simulink model "DEF_IEEE14"  (R2022b)
settings: Solver=FixedStepAuto  StartTime=0  StopTime=15  FixedStep=Ts  RelTol=1e-3
undefined symbols (not defined in the file or in its folder): ApparatusDiscreDamping, ApparatusPara, ApparatusPowerFlow, ApparatusType, Fbase, OtherInputs, Sbase, Ts, Vbase, Wbase, x_e, Ybase, Zbase
libraries: spsGroundLib x22, SimplusGT x22, spsThreePhaseSeriesRLCBranchLib x20, spsThreePhaseParallelRLCBranchLib x14, spsabctoAlphaBetaZeroLib x4, spsThreePhaseTransformerTwoWindingsLib x3, spspowerguiLib x1
settings Model: Creator=y_zhu  LastModifiedBy=yz34218

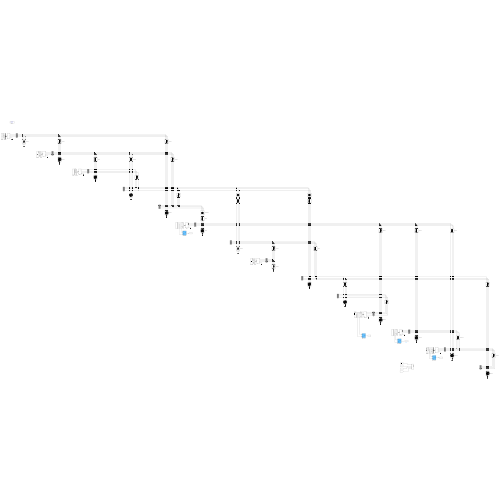
[thumbnail: Simulink's stored preview of the top-level diagram]
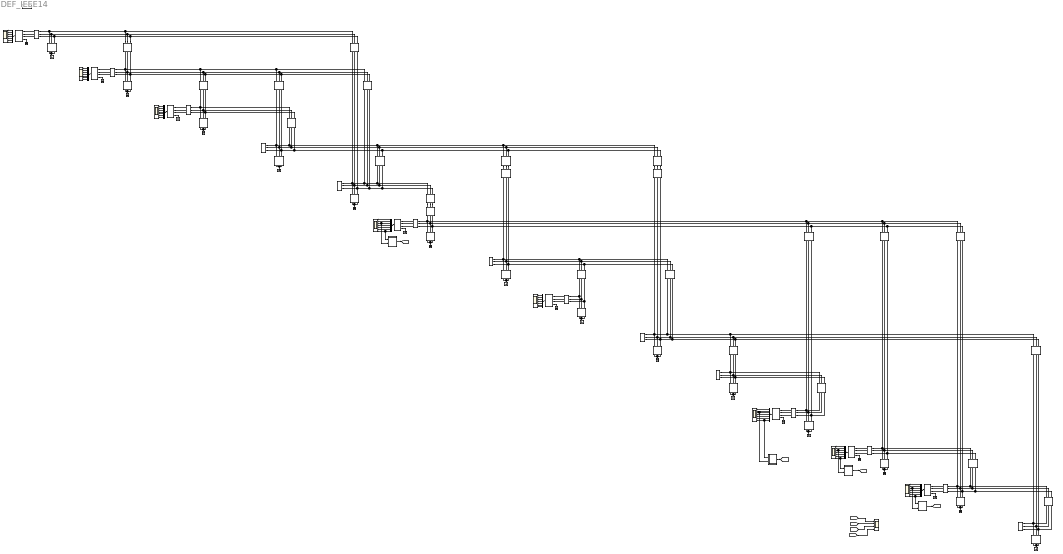
== system DEF_IEEE14 ==
  B-GND{1,4,8,10,14,16,20,23..24,27,29..30,32,34} (14 alike) : spsGroundLib/Ground  LConnTagsString=a
  Branch1-1 : spsThreePhaseParallelRLCBranchLib/Three-Phase Parallel RLC Branch  LConnTagsString=A|B|C  RConnTagsString=A|B|C  BranchType=C  Resistance=(Inf)*Zbase  Inductance=(Inf)*Zbase/Wbase  Capacitance=(0.051)*Ybase/Wbase  Measurements=None
  Branch1-2 : spsThreePhaseSeriesRLCBranchLib/Three-Phase Series RLC Branch  LConnTagsString=A|B|C  RConnTagsString=A|B|C  BranchType=RL  Resistance=(0.01938)*Zbase  Inductance=(0.05917)*Zbase/Wbase  Capacitance=1e-6  Measurements=None
  Branch1-5 : spsThreePhaseSeriesRLCBranchLib/Three-Phase Series RLC Branch  LConnTagsString=A|B|C  RConnTagsString=A|B|C  BranchType=RL  Resistance=(0.05403)*Zbase  Inductance=(0.22304)*Zbase/Wbase  Capacitance=1e-6  Measurements=None
  Branch10-10 : spsThreePhaseParallelRLCBranchLib/Three-Phase Parallel RLC Branch  LConnTagsString=A|B|C  RConnTagsString=A|B|C  BranchType=RLC  Resistance=(12.2907)*Zbase  Inductance=(19.0718)*Zbase/Wbase  Capacitance=(1e-07)*Ybase/Wbase  Measurements=None
  Branch10-11 : spsThreePhaseSeriesRLCBranchLib/Three-Phase Series RLC Branch  LConnTagsString=A|B|C  RConnTagsString=A|B|C  BranchType=RL  Resistance=(0.08205)*Zbase  Inductance=(0.19207)*Zbase/Wbase  Capacitance=1e-6  Measurements=None
  Branch11-11 : spsThreePhaseParallelRLCBranchLib/Three-Phase Parallel RLC Branch  LConnTagsString=A|B|C  RConnTagsString=A|B|C  BranchType=RLC  Resistance=(10.675)*Zbase  Inductance=(62.2711)*Zbase/Wbase  Capacitance=(1e-07)*Ybase/Wbase  Measurements=None
  Branch12-12 : spsThreePhaseParallelRLCBranchLib/Three-Phase Parallel RLC Branch  LConnTagsString=A|B|C  RConnTagsString=A|B|C  BranchType=RLC  Resistance=(6.03)*Zbase  Inductance=(68.9685)*Zbase/Wbase  Capacitance=(1e-07)*Ybase/Wbase  Measurements=None
  Branch12-13 : spsThreePhaseSeriesRLCBranchLib/Three-Phase Series RLC Branch  LConnTagsString=A|B|C  RConnTagsString=A|B|C  BranchType=RL  Resistance=(0.22092)*Zbase  Inductance=(0.19988)*Zbase/Wbase  Capacitance=1e-6  Measurements=None
  Branch13-13 : spsThreePhaseParallelRLCBranchLib/Three-Phase Parallel RLC Branch  LConnTagsString=A|B|C  RConnTagsString=A|B|C  BranchType=RLC  Resistance=(2.6813)*Zbase  Inductance=(18.7232)*Zbase/Wbase  Capacitance=(1.5e-07)*Ybase/Wbase  Measurements=None
  Branch13-14 : spsThreePhaseSeriesRLCBranchLib/Three-Phase Series RLC Branch  LConnTagsString=A|B|C  RConnTagsString=A|B|C  BranchType=RL  Resistance=(0.17093)*Zbase  Inductance=(0.34802)*Zbase/Wbase  Capacitance=1e-6  Measurements=None
  Branch14-14 : spsThreePhaseParallelRLCBranchLib/Three-Phase Parallel RLC Branch  LConnTagsString=A|B|C  RConnTagsString=A|B|C  BranchType=RLC  Resistance=(7.1477)*Zbase  Inductance=(21.3001)*Zbase/Wbase  Capacitance=(1e-07)*Ybase/Wbase  Measurements=None
  Branch2-2 : spsThreePhaseParallelRLCBranchLib/Three-Phase Parallel RLC Branch  LConnTagsString=A|B|C  RConnTagsString=A|B|C  BranchType=RLC  Resistance=(5.0324)*Zbase  Inductance=(8.5986)*Zbase/Wbase  Capacitance=(0.0826)*Ybase/Wbase  Measurements=None
  Branch2-3 : spsThreePhaseSeriesRLCBranchLib/Three-Phase Series RLC Branch  LConnTagsString=A|B|C  RConnTagsString=A|B|C  BranchType=RL  Resistance=(0.04699)*Zbase  Inductance=(0.19797)*Zbase/Wbase  Capacitance=1e-6  Measurements=None
  Branch2-4 : spsThreePhaseSeriesRLCBranchLib/Three-Phase Series RLC Branch  LConnTagsString=A|B|C  RConnTagsString=A|B|C  BranchType=RL  Resistance=(0.05811)*Zbase  Inductance=(0.17632)*Zbase/Wbase  Capacitance=1e-6  Measurements=None
  Branch2-5 : spsThreePhaseSeriesRLCBranchLib/Three-Phase Series RLC Branch  LConnTagsString=A|B|C  RConnTagsString=A|B|C  BranchType=RL  Resistance=(0.05695)*Zbase  Inductance=(0.17388)*Zbase/Wbase  Capacitance=1e-6  Measurements=None
  Branch3-3 : spsThreePhaseParallelRLCBranchLib/Three-Phase Parallel RLC Branch  LConnTagsString=A|B|C  RConnTagsString=A|B|C  BranchType=RLC  Resistance=(1.0829)*Zbase  Inductance=(5.3689)*Zbase/Wbase  Capacitance=(0.0283)*Ybase/Wbase  Measurements=None
  Branch3-4 : spsThreePhaseSeriesRLCBranchLib/Three-Phase Series RLC Branch  LConnTagsString=A|B|C  RConnTagsString=A|B|C  BranchType=RL  Resistance=(0.06701)*Zbase  Inductance=(0.17103)*Zbase/Wbase  Capacitance=1e-6  Measurements=None
  Branch4-4 : spsThreePhaseParallelRLCBranchLib/Three-Phase Parallel RLC Branch  LConnTagsString=A|B|C  RConnTagsString=A|B|C  BranchType=RC  Resistance=(2.1566)*Zbase  Inductance=(Inf)*Zbase/Wbase  Capacitance=(0.061233)*Ybase/Wbase  Measurements=None
  Branch4-5 : spsThreePhaseSeriesRLCBranchLib/Three-Phase Series RLC Branch  LConnTagsString=A|B|C  RConnTagsString=A|B|C  BranchType=RL  Resistance=(0.01335)*Zbase  Inductance=(0.04211)*Zbase/Wbase  Capacitance=1e-6  Measurements=None
  Branch4-7 : spsThreePhaseSeriesRLCBranchLib/Three-Phase Series RLC Branch  LConnTagsString=A|B|C  RConnTagsString=A|B|C  BranchType=RL  Resistance=(1e-07)*Zbase  Inductance=(0.20912)*Zbase/Wbase  Capacitance=1e-6  Measurements=None
  Branch4-9 : spsThreePhaseSeriesRLCBranchLib/Three-Phase Series RLC Branch  LConnTagsString=A|B|C  RConnTagsString=A|B|C  BranchType=RL  Resistance=(1e-07)*Zbase  Inductance=(0.55618)*Zbase/Wbase  Capacitance=1e-6  Measurements=None
  Branch5-5 : spsThreePhaseParallelRLCBranchLib/Three-Phase Parallel RLC Branch  LConnTagsString=A|B|C  RConnTagsString=A|B|C  BranchType=RLC  Resistance=(13.5986)*Zbase  Inductance=(64.5935)*Zbase/Wbase  Capacitance=(0.0419)*Ybase/Wbase  Measurements=None
  Branch5-6 : spsThreePhaseSeriesRLCBranchLib/Three-Phase Series RLC Branch  LConnTagsString=A|B|C  RConnTagsString=A|B|C  BranchType=RL  Resistance=(1e-07)*Zbase  Inductance=(0.25202)*Zbase/Wbase  Capacitance=1e-6  Measurements=None
  Branch6-11 : spsThreePhaseSeriesRLCBranchLib/Three-Phase Series RLC Branch  LConnTagsString=A|B|C  RConnTagsString=A|B|C  BranchType=RL  Resistance=(0.09498)*Zbase  Inductance=(0.1989)*Zbase/Wbase  Capacitance=1e-6  Measurements=None
  Branch6-12 : spsThreePhaseSeriesRLCBranchLib/Three-Phase Series RLC Branch  LConnTagsString=A|B|C  RConnTagsString=A|B|C  BranchType=RL  Resistance=(0.12291)*Zbase  Inductance=(0.25581)*Zbase/Wbase  Capacitance=1e-6  Measurements=None
  Branch6-13 : spsThreePhaseSeriesRLCBranchLib/Three-Phase Series RLC Branch  LConnTagsString=A|B|C  RConnTagsString=A|B|C  BranchType=RL  Resistance=(0.06615)*Zbase  Inductance=(0.13027)*Zbase/Wbase  Capacitance=1e-6  Measurements=None
  Branch6-6 : spsThreePhaseParallelRLCBranchLib/Three-Phase Parallel RLC Branch  LConnTagsString=A|B|C  RConnTagsString=A|B|C  BranchType=RLC  Resistance=(10.2223)*Zbase  Inductance=(15.2653)*Zbase/Wbase  Capacitance=(2e-07)*Ybase/Wbase  Measurements=None
  Branch7-7 : spsThreePhaseParallelRLCBranchLib/Three-Phase Parallel RLC Branch  LConnTagsString=A|B|C  RConnTagsString=A|B|C  BranchType=C  Resistance=(Inf)*Zbase  Inductance=(Inf)*Zbase/Wbase  Capacitance=(1.5e-07)*Ybase/Wbase  Measurements=None
  Branch7-8 : spsThreePhaseSeriesRLCBranchLib/Three-Phase Series RLC Branch  LConnTagsString=A|B|C  RConnTagsString=A|B|C  BranchType=RL  Resistance=(1e-07)*Zbase  Inductance=(0.17615)*Zbase/Wbase  Capacitance=1e-6  Measurements=None
  Branch7-9 : spsThreePhaseSeriesRLCBranchLib/Three-Phase Series RLC Branch  LConnTagsString=A|B|C  RConnTagsString=A|B|C  BranchType=RL  Resistance=(1e-07)*Zbase  Inductance=(0.11001)*Zbase/Wbase  Capacitance=1e-6  Measurements=None
  Branch8-8 : spsThreePhaseParallelRLCBranchLib/Three-Phase Parallel RLC Branch  LConnTagsString=A|B|C  RConnTagsString=A|B|C  BranchType=C  Resistance=(Inf)*Zbase  Inductance=(Inf)*Zbase/Wbase  Capacitance=(5e-08)*Ybase/Wbase  Measurements=None
  Branch9-10 : spsThreePhaseSeriesRLCBranchLib/Three-Phase Series RLC Branch  LConnTagsString=A|B|C  RConnTagsString=A|B|C  BranchType=RL  Resistance=(0.03181)*Zbase  Inductance=(0.0845)*Zbase/Wbase  Capacitance=1e-6  Measurements=None
  Branch9-14 : spsThreePhaseSeriesRLCBranchLib/Three-Phase Series RLC Branch  LConnTagsString=A|B|C  RConnTagsString=A|B|C  BranchType=RL  Resistance=(0.12711)*Zbase  Inductance=(0.27038)*Zbase/Wbase  Capacitance=1e-6  Measurements=None
  Branch9-9 : spsThreePhaseParallelRLCBranchLib/Three-Phase Parallel RLC Branch  LConnTagsString=A|B|C  RConnTagsString=A|B|C  BranchType=RLC  Resistance=(3.7813)*Zbase  Inductance=(6.7198)*Zbase/Wbase  Capacitance=(0.19)*Ybase/Wbase  Measurements=None
  Bus{1..14} (14 alike) : SimplusGT/Three-Phase Bus  Vbase=1  Sbase=1
  D-GND{1..3,6,8,11..13} (8 alike) : spsGroundLib/Ground  LConnTagsString=a
  D-Scope{1..3,6,8,11..13} (8 alike) : Scope  NumInputPorts=7
  DEF_Friction : Subsystem  mask{PowerFlow_App=ApparatusPowerFlow{11}}
      mask prompts: PowerFlow_App "Power Flow"
  DEF_Friction1 : Subsystem  mask{PowerFlow_App=ApparatusPowerFlow{12}}
      mask prompts: PowerFlow_App "Power Flow"
  DEF_Friction2 : Subsystem  mask{PowerFlow_App=ApparatusPowerFlow{13}}
      mask prompts: PowerFlow_App "Power Flow"
  DEF_Friction3 : Subsystem  mask{PowerFlow_App=ApparatusPowerFlow{6}}
      mask prompts: PowerFlow_App "Power Flow"
  DS-Bus{1..3,6,8,11..13} (8 alike) : BusSelector  OutputSignals=v_dq,i_dq,v_abc,i_abc,w,theta,pq
  SM1 : SimplusGT/SynchronousMachineFull_Cyp_SMAVRPSSGOV (dq-Frame System Object)  Ts=Ts  Sbase=Sbase  Vbase=Vbase  Wbase=Wbase  ApparatusType=ApparatusType{1}  ApparatusPara=ApparatusPara{1}  PowerFlow=ApparatusPowerFlow{1}  x0=x_e{1}  OtherInputs=OtherInputs{1}  DiscreMethod=Hybrid Trapezoidal  EnableInsideModification=off  DiscreDampingFlag=on  DiscreDampingValue=ApparatusDiscreDamping{1}  LinearizationTimes=1  DirectFeedthrough=off
  SM2 : SimplusGT/SynchronousMachineFull_Cyp_SMAVRPSSGOV (dq-Frame System Object)  Ts=Ts  Sbase=Sbase  Vbase=Vbase  Wbase=Wbase  ApparatusType=ApparatusType{2}  ApparatusPara=ApparatusPara{2}  PowerFlow=ApparatusPowerFlow{2}  x0=x_e{2}  OtherInputs=OtherInputs{2}  DiscreMethod=Hybrid Trapezoidal  EnableInsideModification=off  DiscreDampingFlag=on  DiscreDampingValue=ApparatusDiscreDamping{2}  LinearizationTimes=1  DirectFeedthrough=off
  SM3 : SimplusGT/SynchronousMachineFull_Cyp_SMAVR (dq-Frame System Object)  Ts=Ts  Sbase=Sbase  Vbase=Vbase  Wbase=Wbase  ApparatusType=ApparatusType{3}  ApparatusPara=ApparatusPara{3}  PowerFlow=ApparatusPowerFlow{3}  x0=x_e{3}  OtherInputs=OtherInputs{3}  DiscreMethod=Hybrid Trapezoidal  EnableInsideModification=off  DiscreDampingFlag=on  DiscreDampingValue=ApparatusDiscreDamping{3}  LinearizationTimes=1  DirectFeedthrough=off
  SM6 : SimplusGT/SynchronousMachineFull_Cyp_SMAVR (dq-Frame System Object)  Ts=Ts  Sbase=Sbase  Vbase=Vbase  Wbase=Wbase  ApparatusType=ApparatusType{6}  ApparatusPara=ApparatusPara{6}  PowerFlow=ApparatusPowerFlow{6}  x0=x_e{6}  OtherInputs=OtherInputs{6}  DiscreMethod=Hybrid Trapezoidal  EnableInsideModification=off  DiscreDampingFlag=on  DiscreDampingValue=ApparatusDiscreDamping{6}  LinearizationTimes=1  DirectFeedthrough=off
  SM8 : SimplusGT/SynchronousMachineFull_Cyp_SMAVR (dq-Frame System Object)  Ts=Ts  Sbase=Sbase  Vbase=Vbase  Wbase=Wbase  ApparatusType=ApparatusType{8}  ApparatusPara=ApparatusPara{8}  PowerFlow=ApparatusPowerFlow{8}  x0=x_e{8}  OtherInputs=OtherInputs{8}  DiscreMethod=Hybrid Trapezoidal  EnableInsideModification=off  DiscreDampingFlag=on  DiscreDampingValue=ApparatusDiscreDamping{8}  LinearizationTimes=1  DirectFeedthrough=off
  Scope : Scope  NumInputPorts=4
  Transformer4-7 : spsThreePhaseTransformerTwoWindingsLib/Three-Phase Transformer (Two Windings)  Winding1Connection=Yg  Winding2Connection=Yg  CoreType=Three single-phase transformers  SetSaturation=off  Hysteresis=off  DataFile='hysteresis'  SetInitialFlux=off  Measurements=None  UNITS=pu  NominalPower=[Sbase, Fbase]  Winding1=[0.978*Vbase, 0, 0]  Winding2=[Vbase, 0, 0]  Rm=1e4  Lm=1e4  L0=0.5  Saturation=[ 0,0 ; 0.0024,1.2 ; 1.0,1.52 ]  InitialFluxes=[ 0.8 , -0.8 , 0.7 ]  BreakLoop=off  DiscreteSolver=Trapezoidal iterative  DataType=off  TransfoNumber=1
  Transformer4-9 : spsThreePhaseTransformerTwoWindingsLib/Three-Phase Transformer (Two Windings)  Winding1Connection=Yg  Winding2Connection=Yg  CoreType=Three single-phase transformers  SetSaturation=off  Hysteresis=off  DataFile='hysteresis'  SetInitialFlux=off  Measurements=None  UNITS=pu  NominalPower=[Sbase, Fbase]  Winding1=[0.969*Vbase, 0, 0]  Winding2=[Vbase, 0, 0]  Rm=1e4  Lm=1e4  L0=0.5  Saturation=[ 0,0 ; 0.0024,1.2 ; 1.0,1.52 ]  InitialFluxes=[ 0.8 , -0.8 , 0.7 ]  BreakLoop=off  DiscreteSolver=Trapezoidal iterative  DataType=off  TransfoNumber=1
  Transformer5-6 : spsThreePhaseTransformerTwoWindingsLib/Three-Phase Transformer (Two Windings)  Winding1Connection=Yg  Winding2Connection=Yg  CoreType=Three single-phase transformers  SetSaturation=off  Hysteresis=off  DataFile='hysteresis'  SetInitialFlux=off  Measurements=None  UNITS=pu  NominalPower=[Sbase, Fbase]  Winding1=[0.932*Vbase, 0, 0]  Winding2=[Vbase, 0, 0]  Rm=1e4  Lm=1e4  L0=0.5  Saturation=[ 0,0 ; 0.0024,1.2 ; 1.0,1.52 ]  InitialFluxes=[ 0.8 , -0.8 , 0.7 ]  BreakLoop=off  DiscreteSolver=Trapezoidal iterative  DataType=off  TransfoNumber=1
  VSI-PLL11 : SimplusGT/Grid-Following Voltage-Source Inverter (dq-Frame System Object)  Ts=Ts  Sbase=Sbase  Vbase=Vbase  Wbase=Wbase  ApparatusType=ApparatusType{11}  ApparatusPara=ApparatusPara{11}  PowerFlow=ApparatusPowerFlow{11}  x0=x_e{11}  OtherInputs=OtherInputs{11}  DiscreMethod=Hybrid Trapezoidal  EnableInsideModification=off  DiscreDampingFlag=on  DiscreDampingValue=ApparatusDiscreDamping{11}  LinearizationTimes=1  DirectFeedthrough=off
  VSI-PLL12 : SimplusGT/Grid-Following Voltage-Source Inverter (dq-Frame System Object)  Ts=Ts  Sbase=Sbase  Vbase=Vbase  Wbase=Wbase  ApparatusType=ApparatusType{12}  ApparatusPara=ApparatusPara{12}  PowerFlow=ApparatusPowerFlow{12}  x0=x_e{12}  OtherInputs=OtherInputs{12}  DiscreMethod=Hybrid Trapezoidal  EnableInsideModification=off  DiscreDampingFlag=on  DiscreDampingValue=ApparatusDiscreDamping{12}  LinearizationTimes=1  DirectFeedthrough=off
  VSI-PLL13 : SimplusGT/Grid-Following Voltage-Source Inverter (dq-Frame System Object)  Ts=Ts  Sbase=Sbase  Vbase=Vbase  Wbase=Wbase  ApparatusType=ApparatusType{13}  ApparatusPara=ApparatusPara{13}  PowerFlow=ApparatusPowerFlow{13}  x0=x_e{13}  OtherInputs=OtherInputs{13}  DiscreMethod=Hybrid Trapezoidal  EnableInsideModification=off  DiscreDampingFlag=on  DiscreDampingValue=ApparatusDiscreDamping{13}  LinearizationTimes=1  DirectFeedthrough=off
  powergui : spspowerguiLib/powergui  Priority=1  SimulationMode=Discrete  SampleTime=Ts  frequency=60  Iterations=50  frequencyindice=0  Pbase=100e6  ErrMax=1e-4  UnitsV=kV  UnitsW=MW  buscounter=0  FunctionMessages=off  echomessages=off  EnableUseOfTLC=off  CurrentSourceSwitches=off  DisableSnubberDevices=off  DisableRonSwitches=off  DisableVfSwitches=off  DisplayEquations=off  AutomaticDiscreteSolvers=off  SolverType=Tustin/Backward Euler (TBE)  Interpol=off  ExternalGateDelay=off  methode=off  Ts=100  x0status=blocks  SPID=on  SwTol=0  HookPort=off  NonlinearTolerance=1e-4  nMaxIteration=100  ContinueOnMaxIteration=off  RestoreLinks=warning  ResistiveCurrentMeasurement=off  Frange=[0:2:500]  Ylog=off  Xlog=on  ShowGrid=off  save=off  variable=ZData  structure=0  ZoomFFT=off  StartTime=0.0  cycles=1  DisplayStyle=1  fundamental=60  FreqAxis=off  MaxFrequency=1000  frequencyindicesteady=1  RmsSteady=1  display=off
  wires:
  SM1/1 -> DS-Bus1/1
  DS-Bus1/1 -> D-Scope1/1  "<v_dq>"
  DS-Bus1/2 -> D-Scope1/2  "<i_dq>"
  DS-Bus1/3 -> D-Scope1/3  "<v_abc>"
  DS-Bus1/4 -> D-Scope1/4  "<i_abc>"
  DS-Bus1/5 -> D-Scope1/5  "<w>"
  DS-Bus1/6 -> D-Scope1/6  "<theta>"
  DS-Bus1/7 -> D-Scope1/7  "<pq>"
  SM2/1 -> DS-Bus2/1
  DS-Bus2/1 -> D-Scope2/1  "<v_dq>"
  DS-Bus2/2 -> D-Scope2/2  "<i_dq>"
  DS-Bus2/3 -> D-Scope2/3  "<v_abc>"
  DS-Bus2/4 -> D-Scope2/4  "<i_abc>"
  DS-Bus2/5 -> D-Scope2/5  "<w>"
  DS-Bus2/6 -> D-Scope2/6  "<theta>"
  DS-Bus2/7 -> D-Scope2/7  "<pq>"
  SM3/1 -> DS-Bus3/1
  DS-Bus3/1 -> D-Scope3/1  "<v_dq>"
  DS-Bus3/2 -> D-Scope3/2  "<i_dq>"
  DS-Bus3/3 -> D-Scope3/3  "<v_abc>"
  DS-Bus3/4 -> D-Scope3/4  "<i_abc>"
  DS-Bus3/5 -> D-Scope3/5  "<w>"
  DS-Bus3/6 -> D-Scope3/6  "<theta>"
  DS-Bus3/7 -> D-Scope3/7  "<pq>"
  SM6/1 -> DS-Bus6/1
  DS-Bus6/1 -> D-Scope6/1  "<v_dq>"
  DS-Bus6/2 -> D-Scope6/2  "<i_dq>"
  DS-Bus6/3 -> DEF_Friction3/2(Vabc), D-Scope6/3  "<v_abc>"
  DS-Bus6/4 -> D-Scope6/4  "<i_abc>"
  DS-Bus6/5 -> D-Scope6/5  "<w>"
  DS-Bus6/6 -> D-Scope6/6  "<theta>"
  DS-Bus6/7 -> DEF_Friction3/1(PQ), D-Scope6/7  "<pq>"
  SM8/1 -> DS-Bus8/1
  DS-Bus8/1 -> D-Scope8/1  "<v_dq>"
  DS-Bus8/2 -> D-Scope8/2  "<i_dq>"
  DS-Bus8/3 -> D-Scope8/3  "<v_abc>"
  DS-Bus8/4 -> D-Scope8/4  "<i_abc>"
  DS-Bus8/5 -> D-Scope8/5  "<w>"
  DS-Bus8/6 -> D-Scope8/6  "<theta>"
  DS-Bus8/7 -> D-Scope8/7  "<pq>"
  VSI-PLL11/1 -> DS-Bus11/1
  DS-Bus11/1 -> D-Scope11/1  "<v_dq>"
  DS-Bus11/2 -> D-Scope11/2  "<i_dq>"
  DS-Bus11/3 -> DEF_Friction/2(Vabc), D-Scope11/3  "<v_abc>"
  DS-Bus11/4 -> D-Scope11/4  "<i_abc>"
  DS-Bus11/5 -> D-Scope11/5  "<w>"
  DS-Bus11/6 -> D-Scope11/6  "<theta>"
  DS-Bus11/7 -> DEF_Friction/1(PQ), D-Scope11/7  "<pq>"
  VSI-PLL12/1 -> DS-Bus12/1
  DS-Bus12/1 -> D-Scope12/1  "<v_dq>"
  DS-Bus12/2 -> D-Scope12/2  "<i_dq>"
  DS-Bus12/3 -> DEF_Friction1/2(Vabc), D-Scope12/3  "<v_abc>"
  DS-Bus12/4 -> D-Scope12/4  "<i_abc>"
  DS-Bus12/5 -> D-Scope12/5  "<w>"
  DS-Bus12/6 -> D-Scope12/6  "<theta>"
  DS-Bus12/7 -> DEF_Friction1/1(PQ), D-Scope12/7  "<pq>"
  VSI-PLL13/1 -> DS-Bus13/1
  DS-Bus13/1 -> D-Scope13/1  "<v_dq>"
  DS-Bus13/2 -> D-Scope13/2  "<i_dq>"
  DS-Bus13/3 -> DEF_Friction2/2(Vabc), D-Scope13/3  "<v_abc>"
  DS-Bus13/4 -> D-Scope13/4  "<i_abc>"
  DS-Bus13/5 -> D-Scope13/5  "<w>"
  DS-Bus13/6 -> D-Scope13/6  "<theta>"
  DS-Bus13/7 -> DEF_Friction2/1(PQ), D-Scope13/7  "<pq>"
  DEF_Friction3/1(DEF) -> [A6]
  DEF_Friction/1(DEF) -> [A11]
  DEF_Friction1/1(DEF) -> [A12]
  DEF_Friction2/1(DEF) -> [A13]
  [A6] -> Scope/1  "A6"
  [A11] -> Scope/2  "A11"
  [A12] -> Scope/3  "A12"
  [A13] -> Scope/4  "A13"
  connections:
  SM1/LConn4 -- D-GND1/LConn1
  SM2/LConn4 -- D-GND2/LConn1
  SM3/LConn4 -- D-GND3/LConn1
  SM6/LConn4 -- D-GND6/LConn1
  SM8/LConn4 -- D-GND8/LConn1
  VSI-PLL11/LConn4 -- D-GND11/LConn1
  VSI-PLL12/LConn4 -- D-GND12/LConn1
  VSI-PLL13/LConn4 -- D-GND13/LConn1
  Branch1-1/RConn1 -- Branch1-1/RConn2 -- Branch1-1/RConn3 -- B-GND1/LConn1
  Branch2-2/RConn1 -- Branch2-2/RConn2 -- Branch2-2/RConn3 -- B-GND4/LConn1
  Branch3-3/RConn1 -- Branch3-3/RConn2 -- Branch3-3/RConn3 -- B-GND8/LConn1
  Branch4-4/RConn1 -- Branch4-4/RConn2 -- Branch4-4/RConn3 -- B-GND10/LConn1
  Branch5-5/RConn1 -- Branch5-5/RConn2 -- Branch5-5/RConn3 -- B-GND14/LConn1
  Branch6-6/RConn1 -- Branch6-6/RConn2 -- Branch6-6/RConn3 -- B-GND16/LConn1
  Branch7-7/RConn1 -- Branch7-7/RConn2 -- Branch7-7/RConn3 -- B-GND20/LConn1
  Branch8-8/RConn1 -- Branch8-8/RConn2 -- Branch8-8/RConn3 -- B-GND23/LConn1
  Branch9-9/RConn1 -- Branch9-9/RConn2 -- Branch9-9/RConn3 -- B-GND24/LConn1
  Branch10-10/RConn1 -- Branch10-10/RConn2 -- Branch10-10/RConn3 -- B-GND27/LConn1
  Branch11-11/RConn1 -- Branch11-11/RConn2 -- Branch11-11/RConn3 -- B-GND29/LConn1
  Branch12-12/RConn1 -- Branch12-12/RConn2 -- Branch12-12/RConn3 -- B-GND30/LConn1
  Branch13-13/RConn1 -- Branch13-13/RConn2 -- Branch13-13/RConn3 -- B-GND32/LConn1
  Branch14-14/RConn1 -- Branch14-14/RConn2 -- Branch14-14/RConn3 -- B-GND34/LConn1
  Branch1-2/RConn1 -- Bus2/RConn1 -- Branch2-2/LConn1 -- Branch2-5/LConn1 -- Branch2-4/LConn1 -- Branch2-3/LConn1
  Branch1-2/RConn2 -- Bus2/RConn2 -- Branch2-2/LConn2 -- Branch2-5/LConn2 -- Branch2-4/LConn2 -- Branch2-3/LConn2
  Branch1-2/RConn3 -- Bus2/RConn3 -- Branch2-2/LConn3 -- Branch2-5/LConn3 -- Branch2-4/LConn3 -- Branch2-3/LConn3
  Branch1-2/LConn1 -- Bus1/RConn1 -- Branch1-1/LConn1 -- Branch1-5/LConn1
  Branch1-2/LConn2 -- Bus1/RConn2 -- Branch1-1/LConn2 -- Branch1-5/LConn2
  Branch1-2/LConn3 -- Bus1/RConn3 -- Branch1-1/LConn3 -- Branch1-5/LConn3
  Branch1-5/RConn1 -- Bus5/RConn1 -- Branch5-5/LConn1 -- Transformer5-6/LConn1 -- Branch4-5/RConn1 -- Branch2-5/RConn1
  Branch1-5/RConn2 -- Bus5/RConn2 -- Branch5-5/LConn2 -- Transformer5-6/LConn2 -- Branch4-5/RConn2 -- Branch2-5/RConn2
  Branch1-5/RConn3 -- Bus5/RConn3 -- Branch5-5/LConn3 -- Transformer5-6/LConn3 -- Branch4-5/RConn3 -- Branch2-5/RConn3
  Branch2-3/RConn1 -- Bus3/RConn1 -- Branch3-3/LConn1 -- Branch3-4/LConn1
  Branch2-3/RConn2 -- Bus3/RConn2 -- Branch3-3/LConn2 -- Branch3-4/LConn2
  Branch2-3/RConn3 -- Bus3/RConn3 -- Branch3-3/LConn3 -- Branch3-4/LConn3
  Branch2-4/RConn1 -- Bus4/RConn1 -- Branch4-4/LConn1 -- Transformer4-9/LConn1 -- Transformer4-7/LConn1 -- Branch4-5/LConn1 -- Branch3-4/RConn1
  Branch2-4/RConn2 -- Bus4/RConn2 -- Branch4-4/LConn2 -- Transformer4-9/LConn2 -- Transformer4-7/LConn2 -- Branch4-5/LConn2 -- Branch3-4/RConn2
  Branch2-4/RConn3 -- Bus4/RConn3 -- Branch4-4/LConn3 -- Transformer4-9/LConn3 -- Transformer4-7/LConn3 -- Branch4-5/LConn3 -- Branch3-4/RConn3
  Branch4-7/RConn1 -- Bus7/RConn1 -- Branch7-7/LConn1 -- Branch7-9/LConn1 -- Branch7-8/LConn1
  Branch4-7/RConn2 -- Bus7/RConn2 -- Branch7-7/LConn2 -- Branch7-9/LConn2 -- Branch7-8/LConn2
  Branch4-7/RConn3 -- Bus7/RConn3 -- Branch7-7/LConn3 -- Branch7-9/LConn3 -- Branch7-8/LConn3
  Transformer4-7/RConn1 -- Branch4-7/LConn1
  Transformer4-7/RConn2 -- Branch4-7/LConn2
  Transformer4-7/RConn3 -- Branch4-7/LConn3
  Branch4-9/RConn1 -- Bus9/RConn1 -- Branch9-9/LConn1 -- Branch9-14/LConn1 -- Branch9-10/LConn1 -- Branch7-9/RConn1
  Branch4-9/RConn2 -- Bus9/RConn2 -- Branch9-9/LConn2 -- Branch9-14/LConn2 -- Branch9-10/LConn2 -- Branch7-9/RConn2
  Branch4-9/RConn3 -- Bus9/RConn3 -- Branch9-9/LConn3 -- Branch9-14/LConn3 -- Branch9-10/LConn3 -- Branch7-9/RConn3
  Transformer4-9/RConn1 -- Branch4-9/LConn1
  Transformer4-9/RConn2 -- Branch4-9/LConn2
  Transformer4-9/RConn3 -- Branch4-9/LConn3
  Branch5-6/RConn1 -- Bus6/RConn1 -- Branch6-6/LConn1 -- Branch6-13/LConn1 -- Branch6-12/LConn1 -- Branch6-11/LConn1
  Branch5-6/RConn2 -- Bus6/RConn2 -- Branch6-6/LConn2 -- Branch6-13/LConn2 -- Branch6-12/LConn2 -- Branch6-11/LConn2
  Branch5-6/RConn3 -- Bus6/RConn3 -- Branch6-6/LConn3 -- Branch6-13/LConn3 -- Branch6-12/LConn3 -- Branch6-11/LConn3
  Transformer5-6/RConn1 -- Branch5-6/LConn1
  Transformer5-6/RConn2 -- Branch5-6/LConn2
  Transformer5-6/RConn3 -- Branch5-6/LConn3
  Branch6-11/RConn1 -- Bus11/RConn1 -- Branch11-11/LConn1 -- Branch10-11/RConn1
  Branch6-11/RConn2 -- Bus11/RConn2 -- Branch11-11/LConn2 -- Branch10-11/RConn2
  Branch6-11/RConn3 -- Bus11/RConn3 -- Branch11-11/LConn3 -- Branch10-11/RConn3
  Branch6-12/RConn1 -- Bus12/RConn1 -- Branch12-12/LConn1 -- Branch12-13/LConn1
  Branch6-12/RConn2 -- Bus12/RConn2 -- Branch12-12/LConn2 -- Branch12-13/LConn2
  Branch6-12/RConn3 -- Bus12/RConn3 -- Branch12-12/LConn3 -- Branch12-13/LConn3
  Branch6-13/RConn1 -- Bus13/RConn1 -- Branch13-13/LConn1 -- Branch13-14/LConn1 -- Branch12-13/RConn1
  Branch6-13/RConn2 -- Bus13/RConn2 -- Branch13-13/LConn2 -- Branch13-14/LConn2 -- Branch12-13/RConn2
  Branch6-13/RConn3 -- Bus13/RConn3 -- Branch13-13/LConn3 -- Branch13-14/LConn3 -- Branch12-13/RConn3
  Branch7-8/RConn1 -- Bus8/RConn1 -- Branch8-8/LConn1
  Branch7-8/RConn2 -- Bus8/RConn2 -- Branch8-8/LConn2
  Branch7-8/RConn3 -- Bus8/RConn3 -- Branch8-8/LConn3
  Branch9-10/RConn1 -- Bus10/RConn1 -- Branch10-10/LConn1 -- Branch10-11/LConn1
  Branch9-10/RConn2 -- Bus10/RConn2 -- Branch10-10/LConn2 -- Branch10-11/LConn2
  Branch9-10/RConn3 -- Bus10/RConn3 -- Branch10-10/LConn3 -- Branch10-11/LConn3
  Branch9-14/RConn1 -- Bus14/RConn1 -- Branch14-14/LConn1 -- Branch13-14/RConn1
  Branch9-14/RConn2 -- Bus14/RConn2 -- Branch14-14/LConn2 -- Branch13-14/RConn2
  Branch9-14/RConn3 -- Bus14/RConn3 -- Branch14-14/LConn3 -- Branch13-14/RConn3
  SM1/LConn1 -- Bus1/LConn1
  SM1/LConn2 -- Bus1/LConn2
  SM1/LConn3 -- Bus1/LConn3
  SM2/LConn1 -- Bus2/LConn1
  SM2/LConn2 -- Bus2/LConn2
  SM2/LConn3 -- Bus2/LConn3
  SM3/LConn1 -- Bus3/LConn1
  SM3/LConn2 -- Bus3/LConn2
  SM3/LConn3 -- Bus3/LConn3
  SM6/LConn1 -- Bus6/LConn1
  SM6/LConn2 -- Bus6/LConn2
  SM6/LConn3 -- Bus6/LConn3
  SM8/LConn1 -- Bus8/LConn1
  SM8/LConn2 -- Bus8/LConn2
  SM8/LConn3 -- Bus8/LConn3
  VSI-PLL11/LConn1 -- Bus11/LConn1
  VSI-PLL11/LConn2 -- Bus11/LConn2
  VSI-PLL11/LConn3 -- Bus11/LConn3
  VSI-PLL12/LConn1 -- Bus12/LConn1
  VSI-PLL12/LConn2 -- Bus12/LConn2
  VSI-PLL12/LConn3 -- Bus12/LConn3
  VSI-PLL13/LConn1 -- Bus13/LConn1
  VSI-PLL13/LConn2 -- Bus13/LConn2
  VSI-PLL13/LConn3 -- Bus13/LConn3

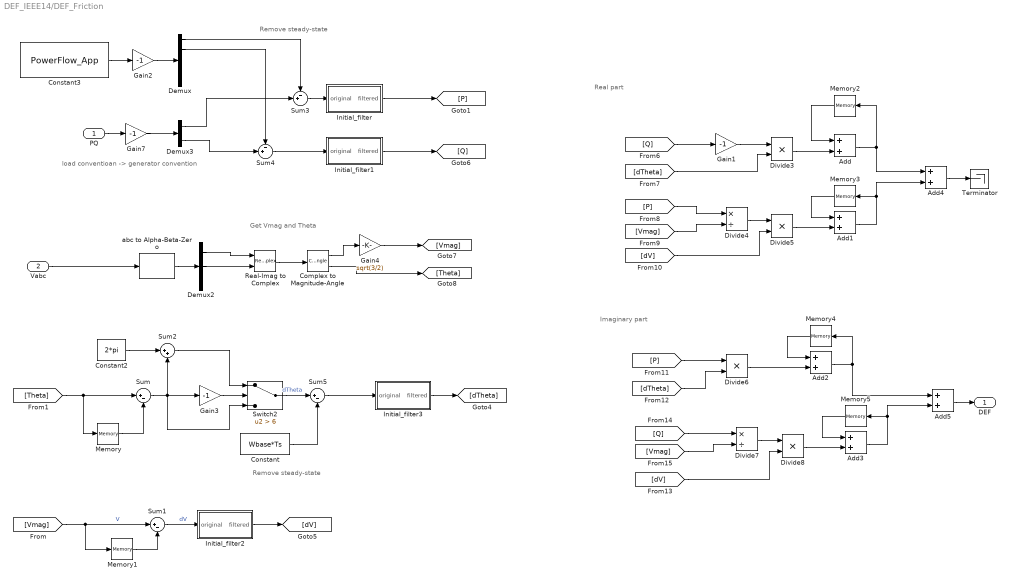
== system DEF_IEEE14/DEF_Friction ==
  note: Real part
  note: Imaginary part
  note: load conventioan -> generator convention
  note: Remove steady-state
  note: Remove steady-state
  note: Get Vmag and Theta
  PQ : Inport
  Vabc : Inport  Port=2
  Add{,1..5} (6 alike) : Sum
  Complex to Magnitude-Angle : ComplexToMagnitudeAngle
  Constant : Constant  Value=Wbase*Ts
  Constant2 : Constant  Value=2*pi
  Constant3 : Constant  Value=PowerFlow_App
  Demux : Demux  Outputs=5
  Demux2 : Demux  Outputs=3
  Demux3 : Demux  Outputs=2
  Divide{3,5..6,8} (4 alike) : Product  Inputs=**
  Divide4 : Product  Inputs=*/
  Divide7 : Product  Inputs=*/
  Gain{1..3,7} (4 alike) : Gain  Gain=-1
  Gain4 : Gain  Gain=sqrt(3/2)
  Initial_filter : Subsystem
  Initial_filter1 : Subsystem
  Initial_filter2 : Subsystem
  Initial_filter3 : Subsystem
  Memory{,1..5} (6 alike) : Memory
  Real-Imag to Complex : RealImagToComplex
  Sum : Sum  Inputs=|+-
  Sum1 : Sum  Inputs=|+-
  Sum2 : Sum  Inputs=|++
  Sum3 : Sum  Inputs=-+|
  Sum4 : Sum  Inputs=-+|
  Sum5 : Sum  Inputs=|+-
  Switch2 : Switch  Criteria=u2 > Threshold  Threshold=6  SaturateOnIntegerOverflow=off  InputSameDT=off
  Terminator : Terminator
  abc to Alpha-Beta-Zero : spsabctoAlphaBetaZeroLib/abc to Alpha-Beta-Zero
  DEF : Outport
  wires:
  [Q] -> Divide7/1
  [Vmag] -> Divide4/2
  Divide3/1 -> Add/2
  [P] -> Divide4/1
  [Q] -> Gain1/1
  Gain1/1 -> Divide3/1
  [dTheta] -> Divide3/2
  [dV] -> Divide5/2
  [P] -> Divide6/1
  Divide4/1 -> Divide5/1
  [dTheta] -> Divide6/2
  [dV] -> Divide8/2
  Divide7/1 -> Divide8/1
  [Vmag] -> Divide7/2
  Memory1/1 -> Sum1/2
  [Vmag] -> Memory1/1, Sum1/1  "V"
  Sum1/1 -> Initial_filter2/1(original)  "dV"
  [Theta] -> Sum/1, Memory/1
  Add/1 -> Memory2/1, Add4/1
  Memory2/1 -> Add/1
  Divide5/1 -> Add1/2
  Add1/1 -> Add4/2, Memory3/1
  Memory3/1 -> Add1/1
  Memory4/1 -> Add2/1
  Add2/1 -> Add5/1, Memory4/1
  Divide6/1 -> Add2/2
  Memory5/1 -> Add3/1
  Add3/1 -> Add5/2, Memory5/1
  Divide8/1 -> Add3/2
  Vabc/1 -> abc to Alpha-Beta-Zero/1
  abc to Alpha-Beta-Zero/1 -> Demux2/1
  Memory/1 -> Sum/2
  Sum/1 -> Gain3/1, Switch2/3, Sum2/2
  Sum2/1 -> Switch2/1
  Constant2/1 -> Sum2/1
  Gain3/1 -> Switch2/2
  Constant3/1 -> Gain2/1
  Sum3/1 -> Initial_filter/1(original)
  Demux/1 -> Sum3/1
  Sum4/1 -> Initial_filter1/1(original)
  Demux/2 -> Sum4/1
  Demux3/1 -> Sum3/2
  Demux3/2 -> Sum4/2
  PQ/1 -> Gain7/1
  Initial_filter/1(filtered) -> [P]
  Initial_filter1/1(filtered) -> [Q]
  Initial_filter2/1(filtered) -> [dV]
  Initial_filter3/1(filtered) -> [dTheta]
  Complex to Magnitude-Angle/2 -> [Theta]
  Gain4/1 -> [Vmag]
  Complex to Magnitude-Angle/1 -> Gain4/1
  Real-Imag to Complex/1 -> Complex to Magnitude-Angle/1
  Demux2/1 -> Real-Imag to Complex/1
  Demux2/2 -> Real-Imag to Complex/2
  Gain2/1 -> Demux/1
  Gain7/1 -> Demux3/1
  Switch2/1 -> Sum5/1  "dTheta"
  Sum5/1 -> Initial_filter3/1(original)
  Constant/1 -> Sum5/2
  Add5/1 -> DEF/1
  Add4/1 -> Terminator/1

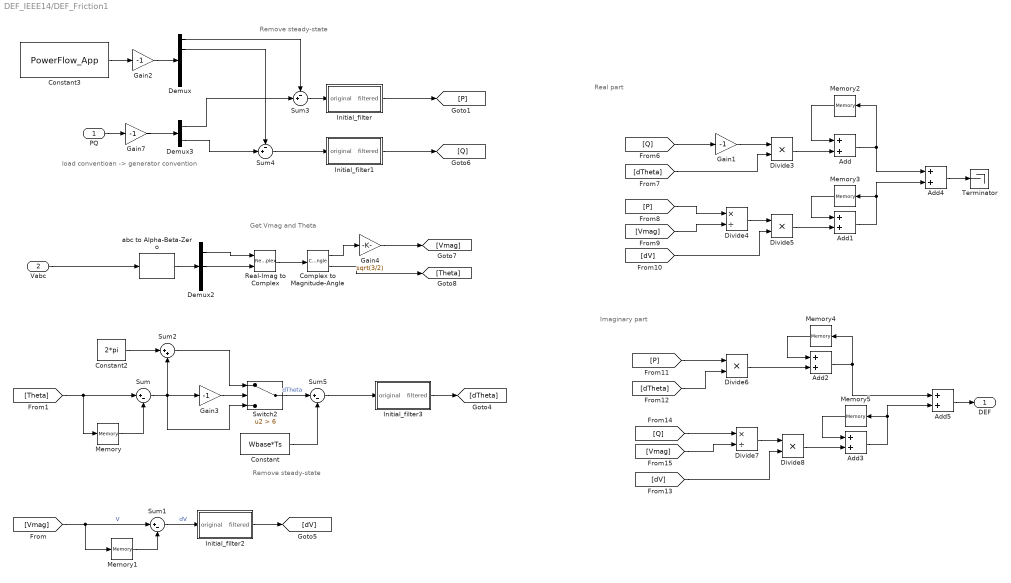
== system DEF_IEEE14/DEF_Friction1 ==
  note: Real part
  note: Imaginary part
  note: load conventioan -> generator convention
  note: Remove steady-state
  note: Remove steady-state
  note: Get Vmag and Theta
  PQ : Inport
  Vabc : Inport  Port=2
  Add{,1..5} (6 alike) : Sum
  Complex to Magnitude-Angle : ComplexToMagnitudeAngle
  Constant : Constant  Value=Wbase*Ts
  Constant2 : Constant  Value=2*pi
  Constant3 : Constant  Value=PowerFlow_App
  Demux : Demux  Outputs=5
  Demux2 : Demux  Outputs=3
  Demux3 : Demux  Outputs=2
  Divide{3,5..6,8} (4 alike) : Product  Inputs=**
  Divide4 : Product  Inputs=*/
  Divide7 : Product  Inputs=*/
  Gain{1..3,7} (4 alike) : Gain  Gain=-1
  Gain4 : Gain  Gain=sqrt(3/2)
  Initial_filter : Subsystem
  Initial_filter1 : Subsystem
  Initial_filter2 : Subsystem
  Initial_filter3 : Subsystem
  Memory{,1..5} (6 alike) : Memory
  Real-Imag to Complex : RealImagToComplex
  Sum : Sum  Inputs=|+-
  Sum1 : Sum  Inputs=|+-
  Sum2 : Sum  Inputs=|++
  Sum3 : Sum  Inputs=-+|
  Sum4 : Sum  Inputs=-+|
  Sum5 : Sum  Inputs=|+-
  Switch2 : Switch  Criteria=u2 > Threshold  Threshold=6  SaturateOnIntegerOverflow=off  InputSameDT=off
  Terminator : Terminator
  abc to Alpha-Beta-Zero : spsabctoAlphaBetaZeroLib/abc to Alpha-Beta-Zero
  DEF : Outport
  wires:
  [Q] -> Divide7/1
  [Vmag] -> Divide4/2
  Divide3/1 -> Add/2
  [P] -> Divide4/1
  [Q] -> Gain1/1
  Gain1/1 -> Divide3/1
  [dTheta] -> Divide3/2
  [dV] -> Divide5/2
  [P] -> Divide6/1
  Divide4/1 -> Divide5/1
  [dTheta] -> Divide6/2
  [dV] -> Divide8/2
  Divide7/1 -> Divide8/1
  [Vmag] -> Divide7/2
  Memory1/1 -> Sum1/2
  [Vmag] -> Memory1/1, Sum1/1  "V"
  Sum1/1 -> Initial_filter2/1(original)  "dV"
  [Theta] -> Sum/1, Memory/1
  Add/1 -> Memory2/1, Add4/1
  Memory2/1 -> Add/1
  Divide5/1 -> Add1/2
  Add1/1 -> Add4/2, Memory3/1
  Memory3/1 -> Add1/1
  Memory4/1 -> Add2/1
  Add2/1 -> Add5/1, Memory4/1
  Divide6/1 -> Add2/2
  Memory5/1 -> Add3/1
  Add3/1 -> Add5/2, Memory5/1
  Divide8/1 -> Add3/2
  Vabc/1 -> abc to Alpha-Beta-Zero/1
  abc to Alpha-Beta-Zero/1 -> Demux2/1
  Memory/1 -> Sum/2
  Sum/1 -> Gain3/1, Switch2/3, Sum2/2
  Sum2/1 -> Switch2/1
  Constant2/1 -> Sum2/1
  Gain3/1 -> Switch2/2
  Constant3/1 -> Gain2/1
  Sum3/1 -> Initial_filter/1(original)
  Demux/1 -> Sum3/1
  Sum4/1 -> Initial_filter1/1(original)
  Demux/2 -> Sum4/1
  Demux3/1 -> Sum3/2
  Demux3/2 -> Sum4/2
  PQ/1 -> Gain7/1
  Initial_filter/1(filtered) -> [P]
  Initial_filter1/1(filtered) -> [Q]
  Initial_filter2/1(filtered) -> [dV]
  Initial_filter3/1(filtered) -> [dTheta]
  Complex to Magnitude-Angle/2 -> [Theta]
  Gain4/1 -> [Vmag]
  Complex to Magnitude-Angle/1 -> Gain4/1
  Real-Imag to Complex/1 -> Complex to Magnitude-Angle/1
  Demux2/1 -> Real-Imag to Complex/1
  Demux2/2 -> Real-Imag to Complex/2
  Gain2/1 -> Demux/1
  Gain7/1 -> Demux3/1
  Switch2/1 -> Sum5/1  "dTheta"
  Sum5/1 -> Initial_filter3/1(original)
  Constant/1 -> Sum5/2
  Add5/1 -> DEF/1
  Add4/1 -> Terminator/1

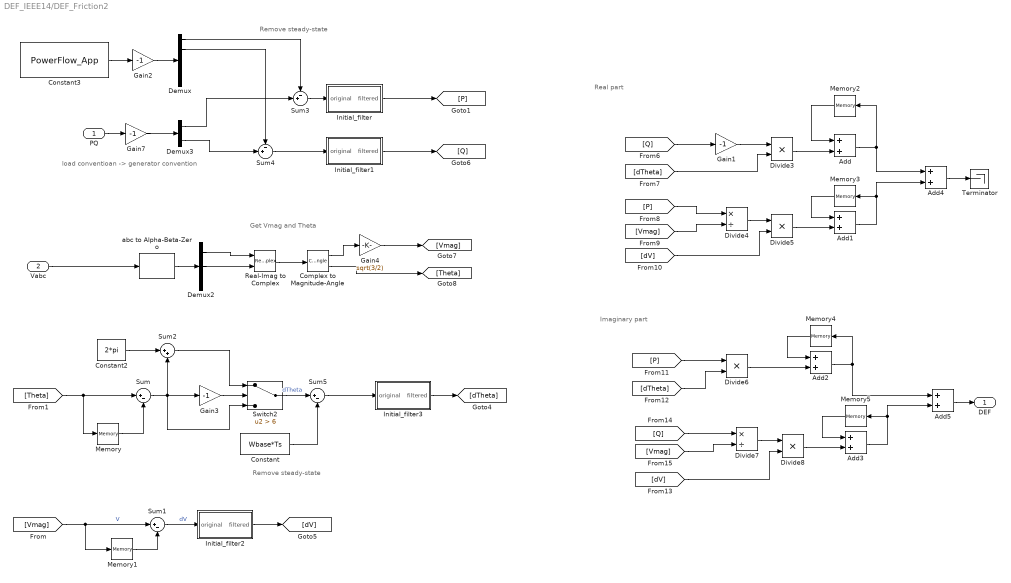
== system DEF_IEEE14/DEF_Friction2 ==
  note: Real part
  note: Imaginary part
  note: load conventioan -> generator convention
  note: Remove steady-state
  note: Remove steady-state
  note: Get Vmag and Theta
  PQ : Inport
  Vabc : Inport  Port=2
  Add{,1..5} (6 alike) : Sum
  Complex to Magnitude-Angle : ComplexToMagnitudeAngle
  Constant : Constant  Value=Wbase*Ts
  Constant2 : Constant  Value=2*pi
  Constant3 : Constant  Value=PowerFlow_App
  Demux : Demux  Outputs=5
  Demux2 : Demux  Outputs=3
  Demux3 : Demux  Outputs=2
  Divide{3,5..6,8} (4 alike) : Product  Inputs=**
  Divide4 : Product  Inputs=*/
  Divide7 : Product  Inputs=*/
  Gain{1..3,7} (4 alike) : Gain  Gain=-1
  Gain4 : Gain  Gain=sqrt(3/2)
  Initial_filter : Subsystem
  Initial_filter1 : Subsystem
  Initial_filter2 : Subsystem
  Initial_filter3 : Subsystem
  Memory{,1..5} (6 alike) : Memory
  Real-Imag to Complex : RealImagToComplex
  Sum : Sum  Inputs=|+-
  Sum1 : Sum  Inputs=|+-
  Sum2 : Sum  Inputs=|++
  Sum3 : Sum  Inputs=-+|
  Sum4 : Sum  Inputs=-+|
  Sum5 : Sum  Inputs=|+-
  Switch2 : Switch  Criteria=u2 > Threshold  Threshold=6  SaturateOnIntegerOverflow=off  InputSameDT=off
  Terminator : Terminator
  abc to Alpha-Beta-Zero : spsabctoAlphaBetaZeroLib/abc to Alpha-Beta-Zero
  DEF : Outport
  wires:
  [Q] -> Divide7/1
  [Vmag] -> Divide4/2
  Divide3/1 -> Add/2
  [P] -> Divide4/1
  [Q] -> Gain1/1
  Gain1/1 -> Divide3/1
  [dTheta] -> Divide3/2
  [dV] -> Divide5/2
  [P] -> Divide6/1
  Divide4/1 -> Divide5/1
  [dTheta] -> Divide6/2
  [dV] -> Divide8/2
  Divide7/1 -> Divide8/1
  [Vmag] -> Divide7/2
  Memory1/1 -> Sum1/2
  [Vmag] -> Memory1/1, Sum1/1  "V"
  Sum1/1 -> Initial_filter2/1(original)  "dV"
  [Theta] -> Sum/1, Memory/1
  Add/1 -> Memory2/1, Add4/1
  Memory2/1 -> Add/1
  Divide5/1 -> Add1/2
  Add1/1 -> Add4/2, Memory3/1
  Memory3/1 -> Add1/1
  Memory4/1 -> Add2/1
  Add2/1 -> Add5/1, Memory4/1
  Divide6/1 -> Add2/2
  Memory5/1 -> Add3/1
  Add3/1 -> Add5/2, Memory5/1
  Divide8/1 -> Add3/2
  Vabc/1 -> abc to Alpha-Beta-Zero/1
  abc to Alpha-Beta-Zero/1 -> Demux2/1
  Memory/1 -> Sum/2
  Sum/1 -> Gain3/1, Switch2/3, Sum2/2
  Sum2/1 -> Switch2/1
  Constant2/1 -> Sum2/1
  Gain3/1 -> Switch2/2
  Constant3/1 -> Gain2/1
  Sum3/1 -> Initial_filter/1(original)
  Demux/1 -> Sum3/1
  Sum4/1 -> Initial_filter1/1(original)
  Demux/2 -> Sum4/1
  Demux3/1 -> Sum3/2
  Demux3/2 -> Sum4/2
  PQ/1 -> Gain7/1
  Initial_filter/1(filtered) -> [P]
  Initial_filter1/1(filtered) -> [Q]
  Initial_filter2/1(filtered) -> [dV]
  Initial_filter3/1(filtered) -> [dTheta]
  Complex to Magnitude-Angle/2 -> [Theta]
  Gain4/1 -> [Vmag]
  Complex to Magnitude-Angle/1 -> Gain4/1
  Real-Imag to Complex/1 -> Complex to Magnitude-Angle/1
  Demux2/1 -> Real-Imag to Complex/1
  Demux2/2 -> Real-Imag to Complex/2
  Gain2/1 -> Demux/1
  Gain7/1 -> Demux3/1
  Switch2/1 -> Sum5/1  "dTheta"
  Sum5/1 -> Initial_filter3/1(original)
  Constant/1 -> Sum5/2
  Add5/1 -> DEF/1
  Add4/1 -> Terminator/1

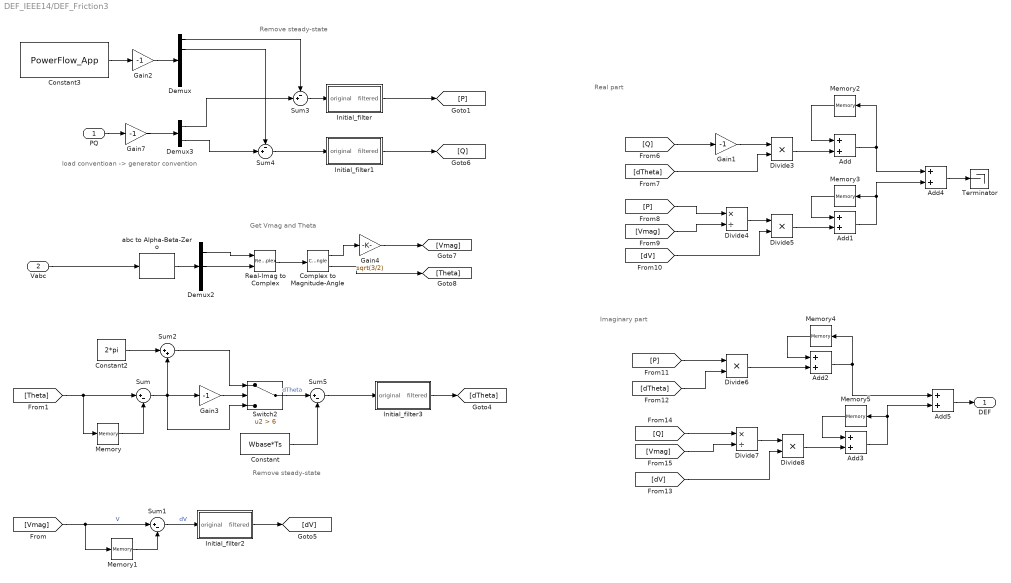
== system DEF_IEEE14/DEF_Friction3 ==
  note: Real part
  note: Imaginary part
  note: load conventioan -> generator convention
  note: Remove steady-state
  note: Remove steady-state
  note: Get Vmag and Theta
  PQ : Inport
  Vabc : Inport  Port=2
  Add{,1..5} (6 alike) : Sum
  Complex to Magnitude-Angle : ComplexToMagnitudeAngle
  Constant : Constant  Value=Wbase*Ts
  Constant2 : Constant  Value=2*pi
  Constant3 : Constant  Value=PowerFlow_App
  Demux : Demux  Outputs=5
  Demux2 : Demux  Outputs=3
  Demux3 : Demux  Outputs=2
  Divide{3,5..6,8} (4 alike) : Product  Inputs=**
  Divide4 : Product  Inputs=*/
  Divide7 : Product  Inputs=*/
  Gain{1..3,7} (4 alike) : Gain  Gain=-1
  Gain4 : Gain  Gain=sqrt(3/2)
  Initial_filter : Subsystem
  Initial_filter1 : Subsystem
  Initial_filter2 : Subsystem
  Initial_filter3 : Subsystem
  Memory{,1..5} (6 alike) : Memory
  Real-Imag to Complex : RealImagToComplex
  Sum : Sum  Inputs=|+-
  Sum1 : Sum  Inputs=|+-
  Sum2 : Sum  Inputs=|++
  Sum3 : Sum  Inputs=-+|
  Sum4 : Sum  Inputs=-+|
  Sum5 : Sum  Inputs=|+-
  Switch2 : Switch  Criteria=u2 > Threshold  Threshold=6  SaturateOnIntegerOverflow=off  InputSameDT=off
  Terminator : Terminator
  abc to Alpha-Beta-Zero : spsabctoAlphaBetaZeroLib/abc to Alpha-Beta-Zero
  DEF : Outport
  wires:
  [Q] -> Divide7/1
  [Vmag] -> Divide4/2
  Divide3/1 -> Add/2
  [P] -> Divide4/1
  [Q] -> Gain1/1
  Gain1/1 -> Divide3/1
  [dTheta] -> Divide3/2
  [dV] -> Divide5/2
  [P] -> Divide6/1
  Divide4/1 -> Divide5/1
  [dTheta] -> Divide6/2
  [dV] -> Divide8/2
  Divide7/1 -> Divide8/1
  [Vmag] -> Divide7/2
  Memory1/1 -> Sum1/2
  [Vmag] -> Memory1/1, Sum1/1  "V"
  Sum1/1 -> Initial_filter2/1(original)  "dV"
  [Theta] -> Sum/1, Memory/1
  Add/1 -> Memory2/1, Add4/1
  Memory2/1 -> Add/1
  Divide5/1 -> Add1/2
  Add1/1 -> Add4/2, Memory3/1
  Memory3/1 -> Add1/1
  Memory4/1 -> Add2/1
  Add2/1 -> Add5/1, Memory4/1
  Divide6/1 -> Add2/2
  Memory5/1 -> Add3/1
  Add3/1 -> Add5/2, Memory5/1
  Divide8/1 -> Add3/2
  Vabc/1 -> abc to Alpha-Beta-Zero/1
  abc to Alpha-Beta-Zero/1 -> Demux2/1
  Memory/1 -> Sum/2
  Sum/1 -> Gain3/1, Switch2/3, Sum2/2
  Sum2/1 -> Switch2/1
  Constant2/1 -> Sum2/1
  Gain3/1 -> Switch2/2
  Constant3/1 -> Gain2/1
  Sum3/1 -> Initial_filter/1(original)
  Demux/1 -> Sum3/1
  Sum4/1 -> Initial_filter1/1(original)
  Demux/2 -> Sum4/1
  Demux3/1 -> Sum3/2
  Demux3/2 -> Sum4/2
  PQ/1 -> Gain7/1
  Initial_filter/1(filtered) -> [P]
  Initial_filter1/1(filtered) -> [Q]
  Initial_filter2/1(filtered) -> [dV]
  Initial_filter3/1(filtered) -> [dTheta]
  Complex to Magnitude-Angle/2 -> [Theta]
  Gain4/1 -> [Vmag]
  Complex to Magnitude-Angle/1 -> Gain4/1
  Real-Imag to Complex/1 -> Complex to Magnitude-Angle/1
  Demux2/1 -> Real-Imag to Complex/1
  Demux2/2 -> Real-Imag to Complex/2
  Gain2/1 -> Demux/1
  Gain7/1 -> Demux3/1
  Switch2/1 -> Sum5/1  "dTheta"
  Sum5/1 -> Initial_filter3/1(original)
  Constant/1 -> Sum5/2
  Add5/1 -> DEF/1
  Add4/1 -> Terminator/1

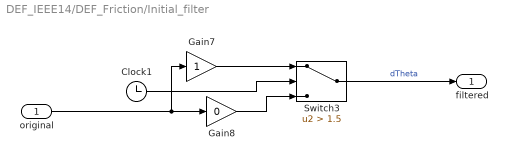
== system DEF_IEEE14/DEF_Friction/Initial_filter ==
  original : Inport
  Clock1 : Clock
  Gain7 : Gain
  Gain8 : Gain  Gain=0
  Switch3 : Switch  Criteria=u2 > Threshold  Threshold=1.5  SaturateOnIntegerOverflow=off  InputSameDT=off
  filtered : Outport
  wires:
  Switch3/1 -> filtered/1  "dTheta"
  original/1 -> Gain8/1, Gain7/1
  Gain7/1 -> Switch3/1
  Gain8/1 -> Switch3/3
  Clock1/1 -> Switch3/2

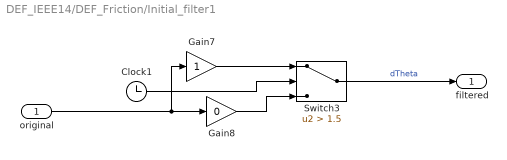
== system DEF_IEEE14/DEF_Friction/Initial_filter1 ==
  original : Inport
  Clock1 : Clock
  Gain7 : Gain
  Gain8 : Gain  Gain=0
  Switch3 : Switch  Criteria=u2 > Threshold  Threshold=1.5  SaturateOnIntegerOverflow=off  InputSameDT=off
  filtered : Outport
  wires:
  Switch3/1 -> filtered/1  "dTheta"
  original/1 -> Gain8/1, Gain7/1
  Gain7/1 -> Switch3/1
  Gain8/1 -> Switch3/3
  Clock1/1 -> Switch3/2

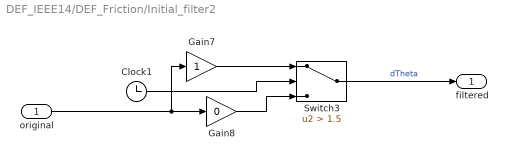
== system DEF_IEEE14/DEF_Friction/Initial_filter2 ==
  original : Inport
  Clock1 : Clock
  Gain7 : Gain
  Gain8 : Gain  Gain=0
  Switch3 : Switch  Criteria=u2 > Threshold  Threshold=1.5  SaturateOnIntegerOverflow=off  InputSameDT=off
  filtered : Outport
  wires:
  Switch3/1 -> filtered/1  "dTheta"
  original/1 -> Gain8/1, Gain7/1
  Gain7/1 -> Switch3/1
  Gain8/1 -> Switch3/3
  Clock1/1 -> Switch3/2

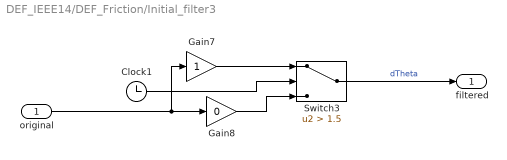
== system DEF_IEEE14/DEF_Friction/Initial_filter3 ==
  original : Inport
  Clock1 : Clock
  Gain7 : Gain
  Gain8 : Gain  Gain=0
  Switch3 : Switch  Criteria=u2 > Threshold  Threshold=1.5  SaturateOnIntegerOverflow=off  InputSameDT=off
  filtered : Outport
  wires:
  Switch3/1 -> filtered/1  "dTheta"
  original/1 -> Gain8/1, Gain7/1
  Gain7/1 -> Switch3/1
  Gain8/1 -> Switch3/3
  Clock1/1 -> Switch3/2

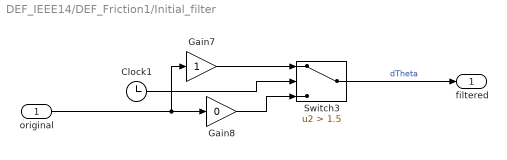
== system DEF_IEEE14/DEF_Friction1/Initial_filter ==
  original : Inport
  Clock1 : Clock
  Gain7 : Gain
  Gain8 : Gain  Gain=0
  Switch3 : Switch  Criteria=u2 > Threshold  Threshold=1.5  SaturateOnIntegerOverflow=off  InputSameDT=off
  filtered : Outport
  wires:
  Switch3/1 -> filtered/1  "dTheta"
  original/1 -> Gain8/1, Gain7/1
  Gain7/1 -> Switch3/1
  Gain8/1 -> Switch3/3
  Clock1/1 -> Switch3/2

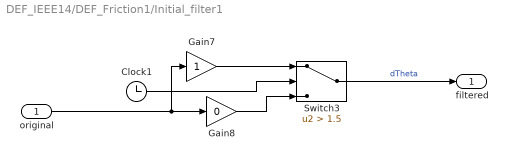
== system DEF_IEEE14/DEF_Friction1/Initial_filter1 ==
  original : Inport
  Clock1 : Clock
  Gain7 : Gain
  Gain8 : Gain  Gain=0
  Switch3 : Switch  Criteria=u2 > Threshold  Threshold=1.5  SaturateOnIntegerOverflow=off  InputSameDT=off
  filtered : Outport
  wires:
  Switch3/1 -> filtered/1  "dTheta"
  original/1 -> Gain8/1, Gain7/1
  Gain7/1 -> Switch3/1
  Gain8/1 -> Switch3/3
  Clock1/1 -> Switch3/2

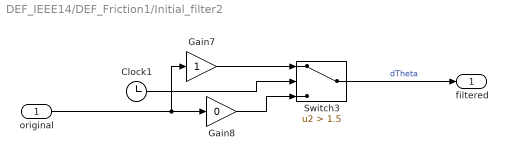
== system DEF_IEEE14/DEF_Friction1/Initial_filter2 ==
  original : Inport
  Clock1 : Clock
  Gain7 : Gain
  Gain8 : Gain  Gain=0
  Switch3 : Switch  Criteria=u2 > Threshold  Threshold=1.5  SaturateOnIntegerOverflow=off  InputSameDT=off
  filtered : Outport
  wires:
  Switch3/1 -> filtered/1  "dTheta"
  original/1 -> Gain8/1, Gain7/1
  Gain7/1 -> Switch3/1
  Gain8/1 -> Switch3/3
  Clock1/1 -> Switch3/2

== system DEF_IEEE14/DEF_Friction1/Initial_filter3 ==
  original : Inport
  Clock1 : Clock
  Gain7 : Gain
  Gain8 : Gain  Gain=0
  Switch3 : Switch  Criteria=u2 > Threshold  Threshold=1.5  SaturateOnIntegerOverflow=off  InputSameDT=off
  filtered : Outport
  wires:
  Switch3/1 -> filtered/1  "dTheta"
  original/1 -> Gain8/1, Gain7/1
  Gain7/1 -> Switch3/1
  Gain8/1 -> Switch3/3
  Clock1/1 -> Switch3/2

== system DEF_IEEE14/DEF_Friction2/Initial_filter ==
  original : Inport
  Clock1 : Clock
  Gain7 : Gain
  Gain8 : Gain  Gain=0
  Switch3 : Switch  Criteria=u2 > Threshold  Threshold=1.5  SaturateOnIntegerOverflow=off  InputSameDT=off
  filtered : Outport
  wires:
  Switch3/1 -> filtered/1  "dTheta"
  original/1 -> Gain8/1, Gain7/1
  Gain7/1 -> Switch3/1
  Gain8/1 -> Switch3/3
  Clock1/1 -> Switch3/2

== system DEF_IEEE14/DEF_Friction2/Initial_filter1 ==
  original : Inport
  Clock1 : Clock
  Gain7 : Gain
  Gain8 : Gain  Gain=0
  Switch3 : Switch  Criteria=u2 > Threshold  Threshold=1.5  SaturateOnIntegerOverflow=off  InputSameDT=off
  filtered : Outport
  wires:
  Switch3/1 -> filtered/1  "dTheta"
  original/1 -> Gain8/1, Gain7/1
  Gain7/1 -> Switch3/1
  Gain8/1 -> Switch3/3
  Clock1/1 -> Switch3/2

== system DEF_IEEE14/DEF_Friction2/Initial_filter2 ==
  original : Inport
  Clock1 : Clock
  Gain7 : Gain
  Gain8 : Gain  Gain=0
  Switch3 : Switch  Criteria=u2 > Threshold  Threshold=1.5  SaturateOnIntegerOverflow=off  InputSameDT=off
  filtered : Outport
  wires:
  Switch3/1 -> filtered/1  "dTheta"
  original/1 -> Gain8/1, Gain7/1
  Gain7/1 -> Switch3/1
  Gain8/1 -> Switch3/3
  Clock1/1 -> Switch3/2

== system DEF_IEEE14/DEF_Friction2/Initial_filter3 ==
  original : Inport
  Clock1 : Clock
  Gain7 : Gain
  Gain8 : Gain  Gain=0
  Switch3 : Switch  Criteria=u2 > Threshold  Threshold=1.5  SaturateOnIntegerOverflow=off  InputSameDT=off
  filtered : Outport
  wires:
  Switch3/1 -> filtered/1  "dTheta"
  original/1 -> Gain8/1, Gain7/1
  Gain7/1 -> Switch3/1
  Gain8/1 -> Switch3/3
  Clock1/1 -> Switch3/2

== system DEF_IEEE14/DEF_Friction3/Initial_filter ==
  original : Inport
  Clock1 : Clock
  Gain7 : Gain
  Gain8 : Gain  Gain=0
  Switch3 : Switch  Criteria=u2 > Threshold  Threshold=1.5  SaturateOnIntegerOverflow=off  InputSameDT=off
  filtered : Outport
  wires:
  Switch3/1 -> filtered/1  "dTheta"
  original/1 -> Gain8/1, Gain7/1
  Gain7/1 -> Switch3/1
  Gain8/1 -> Switch3/3
  Clock1/1 -> Switch3/2

== system DEF_IEEE14/DEF_Friction3/Initial_filter1 ==
  original : Inport
  Clock1 : Clock
  Gain7 : Gain
  Gain8 : Gain  Gain=0
  Switch3 : Switch  Criteria=u2 > Threshold  Threshold=1.5  SaturateOnIntegerOverflow=off  InputSameDT=off
  filtered : Outport
  wires:
  Switch3/1 -> filtered/1  "dTheta"
  original/1 -> Gain8/1, Gain7/1
  Gain7/1 -> Switch3/1
  Gain8/1 -> Switch3/3
  Clock1/1 -> Switch3/2

== system DEF_IEEE14/DEF_Friction3/Initial_filter2 ==
  original : Inport
  Clock1 : Clock
  Gain7 : Gain
  Gain8 : Gain  Gain=0
  Switch3 : Switch  Criteria=u2 > Threshold  Threshold=1.5  SaturateOnIntegerOverflow=off  InputSameDT=off
  filtered : Outport
  wires:
  Switch3/1 -> filtered/1  "dTheta"
  original/1 -> Gain8/1, Gain7/1
  Gain7/1 -> Switch3/1
  Gain8/1 -> Switch3/3
  Clock1/1 -> Switch3/2

== system DEF_IEEE14/DEF_Friction3/Initial_filter3 ==
  original : Inport
  Clock1 : Clock
  Gain7 : Gain
  Gain8 : Gain  Gain=0
  Switch3 : Switch  Criteria=u2 > Threshold  Threshold=1.5  SaturateOnIntegerOverflow=off  InputSameDT=off
  filtered : Outport
  wires:
  Switch3/1 -> filtered/1  "dTheta"
  original/1 -> Gain8/1, Gain7/1
  Gain7/1 -> Switch3/1
  Gain8/1 -> Switch3/3
  Clock1/1 -> Switch3/2
